simulink model "Core1MC"  (R2025a)
settings: Solver=FixedStepDiscrete  StartTime=0.0  StopTime=10.0  RelTol=1e-3
settings Model: Creator=mfussi  LastModifiedBy=mfussi
settings OptimizationCC: DefaultParameterBehavior=Inlined  EnhancedBackFolding=on  PassReuseOutputArgsAs=Individual arguments  ZeroExternalMemoryAtStartup=off  ZeroInternalMemoryAtStartup=off  OptimizeBlockOrder=speed  DifferentSizesBufferReuse=on  OptimizationCustomize=off  EfficientTunableParamExpr=on
settings DebuggingCC: ParameterTunabilityLossMsg=error
settings SFSimCC: MATLABDynamicMemAlloc=off
settings RTWCC: SystemTargetFile=ert.tlc  TemplateMakefile=ert_default_tmf  Description=Embedded Coder
settings CodeAppCC: ForceParamTrailComments=on  IgnoreCustomStorageClasses=off  OperatorAnnotations=on  SimulinkDataObjDesc=on  SFDataObjDesc=on  InsertBlockDesc=on
settings ERTTargetCC: ExtModeTransport=0.0  ExtModeStaticAlloc=off  ExtModeMexFile=ext_comm  ExtModeIntrfLevel=Level1  ERTCustomFileTemplate=example_file_process.tlc  TargetLangStandard=C99 (ISO)  GenerateSampleERTMain=on

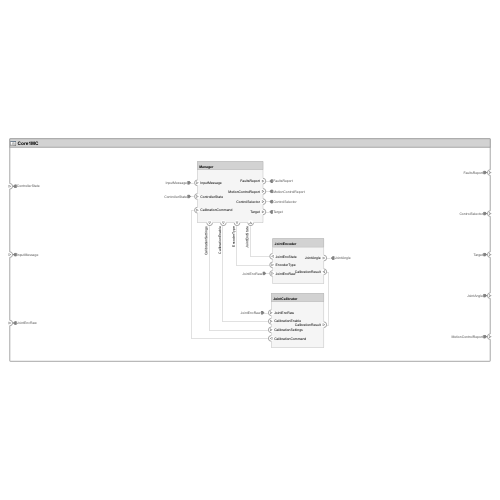
[thumbnail: Simulink's stored preview of the top-level diagram]
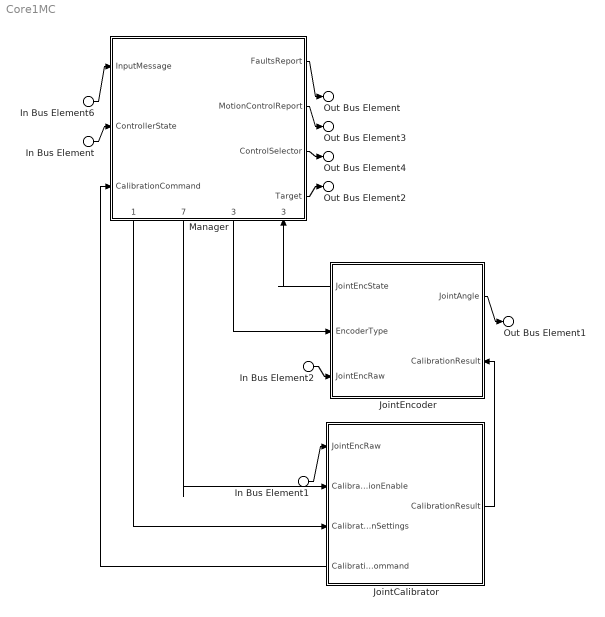
== system Core1MC ==
  In Bus Element : Inport  PortName=ControllerState
  In Bus Element6 : Inport  Port=2  PortName=InputMessage
  In Bus Element2 : Inport  Port=3  PortName=JointEncRaw
  In Bus Element1 : Inport  Port=3  PortName=JointEncRaw
  JointCalibrator : Subsystem
      settings: PortSchema="{\"entries\":[{\"content\":{\"headerSize\":26,\"margin\":15,\"minimumSpacing\":25,\"sides\":[{\"content\":{\"connectorIds\":[\"In3\",\"In1\",\"In2\",\"Out2\"]},\"type\":\"ConnectorPlacement.EquallySpacedRectSide\",\"uuid\":\"01a9f67f-de41-4770-8c99-b8ecc5be53ce\"},{\"content\":{\"connectorIds\":[\"Out1\"],\"side\":\"RIGHT\"},\"type\":\"ConnectorPlacement.EquallySpacedRectSide\",\"uuid\":\"bf951eb2-be85-4331-ab1b-e1ec4c58de10\"},{\"content\":{\"side\":\"TOP\"},\"type\":\"ConnectorPlacement.EquallySpacedRectSide\",\"uuid\":\"bda0090a-3dbc-4c35-be89-fb46a9401bc0\"},{\"content\":{\"side\":\"BOTTOM\"},\"type\":\"ConnectorPlacement.EquallySpacedRectSide\",\"uuid\":\"ec3dea10-cab4-440e-89eb-654eef2537c3\"}]},\"type\":\"ConnectorPlacement.EquallySpacedConnector\",\"uuid\":\"c83d3565-87fc-4d8e-ad9f-6c471e7c3840\"}],\"packageUris\":[\"http://schema.mathworks.com/mf0/Connector/R2020b\"],\"version\":\"1.0\"}"
  JointEncoder : Subsystem
      settings: PortSchema="{\"entries\":[{\"content\":{\"headerSize\":26,\"margin\":15,\"minimumSpacing\":25,\"sides\":[{\"content\":{\"connectorIds\":[\"Out1\",\"In1\",\"In3\"]},\"type\":\"ConnectorPlacement.EquallySpacedRectSide\",\"uuid\":\"01a9f67f-de41-4770-8c99-b8ecc5be53ce\"},{\"content\":{\"connectorIds\":[\"Out2\",\"In2\"],\"side\":\"RIGHT\"},\"type\":\"ConnectorPlacement.EquallySpacedRectSide\",\"uuid\":\"bf951eb2-be85-4331-ab1b-e1ec4c58de10\"},{\"content\":{\"side\":\"TOP\"},\"type\":\"ConnectorPlacement.EquallySpacedRectSide\",\"uuid\":\"bda0090a-3dbc-4c35-be89-fb46a9401bc0\"},{\"content\":{\"side\":\"BOTTOM\"},\"type\":\"ConnectorPlacement.EquallySpacedRectSide\",\"uuid\":\"08402c68-e81a-4e51-a9bb-186315986595\"}]},\"type\":\"ConnectorPlacement.EquallySpacedConnector\",\"uuid\":\"c83d3565-87fc-4d8e-ad9f-6c471e7c3840\"}],\"packageUris\":[\"http://schema.mathworks.com/mf0/Connector/R2020b\"],\"version\":\"1.0\"}"
  Manager : Subsystem
      settings: PortSchema="{\"entries\":[{\"content\":{\"headerSize\":26,\"margin\":15,\"minimumSpacing\":25,\"sides\":[{\"content\":{\"connectorIds\":[\"In1\",\"In4\",\"In2\"]},\"type\":\"ConnectorPlacement.EquallySpacedRectSide\",\"uuid\":\"8e6109ac-b489-4864-8b2b-7ebf0beccfe4\"},{\"content\":{\"connectorIds\":[\"Out2\",\"Out5\",\"Out4\",\"Out6\"],\"side\":\"RIGHT\"},\"type\":\"ConnectorPlacement.EquallySpacedRectSide\",\"uuid\":\"71828a7e-6b05-4f57-abc1-6f865453b9f6\"},{\"content\":{\"side\":\"TOP\"},\"type\":\"ConnectorPlacement.EquallySpacedRectSide\",\"uuid\":\"bfeeaaf9-6170-4b48-807f-b679c72692dc\"},{\"content\":{\"connectorIds\":[\"Out1\",\"Out7\",\"Out3\",\"In3\"],\"side\":\"BOTTOM\"},\"type\":\"ConnectorPlacement.EquallySpacedRectSide\",\"uuid\":\"8d96d7f2-73a1-4d5a-99fb-90680abef3dc\"}]},\"type\":\"ConnectorPlacement.EquallySpacedConnector\",\"uuid\":\"352ed8e9-1880-4bea-97e7-a2aba6f573a0\"}],\"packageUris\":[\"http://schema.mathworks.com/mf0/Connector/R2020b\"],\"version\":\"1.0\"}"
  Out Bus Element : Outport  PortName=FaultsReport
  Out Bus Element4 : Outport  Port=2  PortName=ControlSelector
  Out Bus Element2 : Outport  Port=3  PortName=Target
  Out Bus Element1 : Outport  Port=4  PortName=JointAngle
  Out Bus Element3 : Outport  Port=5  PortName=MotionControlReport
  wires:
  Manager/7(CalibrationEnable) -> JointCalibrator/1(CalibrationEnable)
  Manager/6(Target) -> Out Bus Element2/1
  Manager/1(CalibrationSettings) -> JointCalibrator/2(CalibrationSettings)
  JointEncoder/2(JointAngle) -> Out Bus Element1/1
  In Bus Element2/1 -> JointEncoder/3(JointEncRaw)
  Manager/2(FaultsReport) -> Out Bus Element/1
  JointCalibrator/2(CalibrationCommand) -> Manager/2(CalibrationCommand)
  Manager/5(MotionControlReport) -> Out Bus Element3/1
  In Bus Element1/1 -> JointCalibrator/3(JointEncRaw)
  Manager/3(EncoderType) -> JointEncoder/1(EncoderType)
  In Bus Element6/1 -> Manager/1(InputMessage)
  JointCalibrator/1(CalibrationResult) -> JointEncoder/2(CalibrationResult)
  JointEncoder/1(JointEncState) -> Manager/3(JointEncState)
  Manager/4(ControlSelector) -> Out Bus Element4/1
  In Bus Element/1 -> Manager/4(ControllerState)

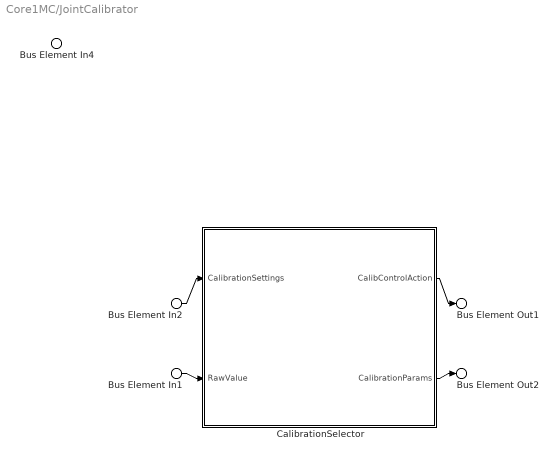
== system Core1MC/JointCalibrator ==
  Bus Element In4 : Inport  PortName=CalibrationEnable
  Bus Element In2 : Inport  Port=2  PortName=CalibrationSettings
  Bus Element In1 : Inport  Port=3  PortName=JointEncRaw
  CalibrationSelector : Subsystem
      settings: PortSchema="{\"entries\":[{\"content\":{\"headerSize\":26,\"margin\":15,\"minimumSpacing\":25,\"sides\":[{\"content\":{\"connectorIds\":[\"In1\",\"In2\"]},\"type\":\"ConnectorPlacement.EquallySpacedRectSide\",\"uuid\":\"8e6109ac-b489-4864-8b2b-7ebf0beccfe4\"},{\"content\":{\"connectorIds\":[\"Out1\",\"Out2\"],\"side\":\"RIGHT\"},\"type\":\"ConnectorPlacement.EquallySpacedRectSide\",\"uuid\":\"71828a7e-6b05-4f57-abc1-6f865453b9f6\"},{\"content\":{\"side\":\"TOP\"},\"type\":\"ConnectorPlacement.EquallySpacedRectSide\",\"uuid\":\"bfeeaaf9-6170-4b48-807f-b679c72692dc\"},{\"content\":{\"side\":\"BOTTOM\"},\"type\":\"ConnectorPlacement.EquallySpacedRectSide\",\"uuid\":\"25c92704-7839-4043-9d29-39ffe7db8a81\"}]},\"type\":\"ConnectorPlacement.EquallySpacedConnector\",\"uuid\":\"352ed8e9-1880-4bea-97e7-a2aba6f573a0\"}],\"packageUris\":[\"http://schema.mathworks.com/mf0/Connector/R2020b\"],\"version\":\"1.0\"}"
  Bus Element Out2 : Outport  PortName=CalibrationResult
  Bus Element Out1 : Outport  Port=2  PortName=CalibrationCommand
  wires:
  Bus Element In2/1 -> CalibrationSelector/1(CalibrationSettings)
  CalibrationSelector/2(CalibrationParams) -> Bus Element Out2/1
  Bus Element In1/1 -> CalibrationSelector/2(RawValue)
  CalibrationSelector/1(CalibControlAction) -> Bus Element Out1/1

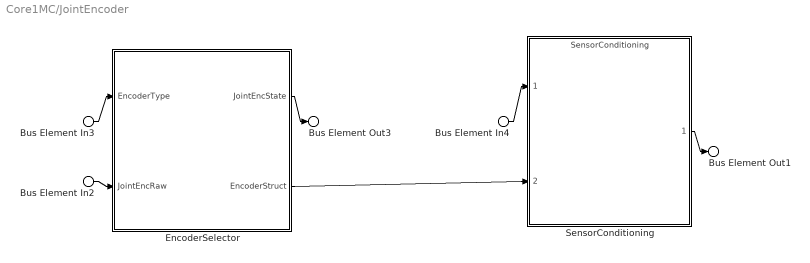
== system Core1MC/JointEncoder ==
  Bus Element In3 : Inport  PortName=EncoderType
  Bus Element In4 : Inport  Port=2  PortName=CalibrationResult
  Bus Element In2 : Inport  Port=3  PortName=JointEncRaw
  EncoderSelector : Subsystem
      settings: PortSchema="{\"entries\":[{\"content\":{\"headerSize\":26,\"margin\":15,\"minimumSpacing\":25,\"sides\":[{\"content\":{\"connectorIds\":[\"In1\",\"In2\"]},\"type\":\"ConnectorPlacement.EquallySpacedRectSide\",\"uuid\":\"8f52fc44-033b-42c5-ba74-e10c3c4c9620\"},{\"content\":{\"connectorIds\":[\"Out1\",\"Out2\"],\"side\":\"RIGHT\"},\"type\":\"ConnectorPlacement.EquallySpacedRectSide\",\"uuid\":\"3378411c-333a-4ac7-97cd-fc73e032020d\"},{\"content\":{\"side\":\"TOP\"},\"type\":\"ConnectorPlacement.EquallySpacedRectSide\",\"uuid\":\"71f34e7e-b8af-4493-b4da-76896ccc3fbc\"}]},\"type\":\"ConnectorPlacement.EquallySpacedConnector\",\"uuid\":\"3896a3b2-2849-4eb4-a68e-00b6690583b8\"}],\"packageUris\":[\"http://schema.mathworks.com/mf0/Connector/R2020b\"],\"version\":\"1.0\"}"
  SensorConditioning : ModelReference  ModelNameDialog=SensorConditioning.slx  SimulationMode=Normal  ScheduleRates=on  ModelReferenceVersion=1.2
      settings: PortSchema="{\"entries\":[{\"content\":{\"headerSize\":38,\"margin\":15,\"minimumSpacing\":25,\"sides\":[{\"content\":{\"connectorIds\":[\"In1\",\"In2\"]},\"type\":\"ConnectorPlacement.EquallySpacedRectSide\",\"uuid\":\"6d6857fa-f5c9-43b4-a306-0920391a2fd0\"},{\"content\":{\"connectorIds\":[\"Out1\"],\"side\":\"RIGHT\"},\"type\":\"ConnectorPlacement.EquallySpacedRectSide\",\"uuid\":\"4567897e-6982-4f2c-af43-5ed4bc8792a2\"},{\"content\":{\"side\":\"TOP\"},\"type\":\"ConnectorPlacement.EquallySpacedRectSide\",\"uuid\":\"b9101744-fe35-433d-bb4c-e7449aefab81\"}]},\"type\":\"ConnectorPlacement.EquallySpacedConnector\",\"uuid\":\"96c92cf5-557b-4ff0-b6b4-f2ae6063b6b3\"}],\"packageUris\":[\"http://schema.mathworks.com/mf0/Connector/R2020b\"],\"version\":\"1.0\"}"
  Bus Element Out3 : Outport  PortName=JointEncState
  Bus Element Out1 : Outport  Port=2  PortName=JointAngle
  wires:
  Bus Element In3/1 -> EncoderSelector/1(EncoderType)
  SensorConditioning/1 -> Bus Element Out1/1
  Bus Element In4/1 -> SensorConditioning/1
  Bus Element In2/1 -> EncoderSelector/2(JointEncRaw)
  EncoderSelector/2(EncoderStruct) -> SensorConditioning/2
  EncoderSelector/1(JointEncState) -> Bus Element Out3/1

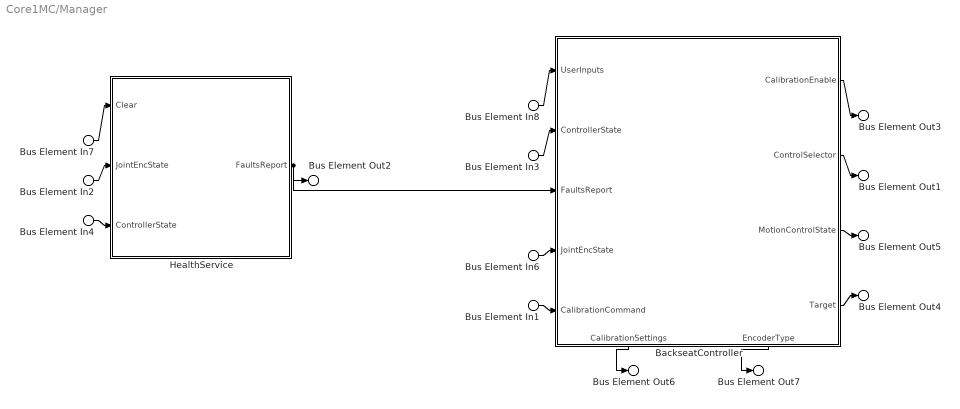
== system Core1MC/Manager ==
  Bus Element In8 : Inport  PortName=InputMessage
  Bus Element In7 : Inport  PortName=InputMessage  Element=ClearFaults
  Bus Element In1 : Inport  Port=2  PortName=CalibrationCommand
  Bus Element In2 : Inport  Port=3  PortName=JointEncState
  Bus Element In6 : Inport  Port=3  PortName=JointEncState
  Bus Element In3 : Inport  Port=4  PortName=ControllerState
  Bus Element In4 : Inport  Port=4  PortName=ControllerState
  "BackseatController   " : Subsystem
      settings: PortSchema="{\"entries\":[{\"content\":{\"headerSize\":26,\"margin\":15,\"minimumSpacing\":25,\"sides\":[{\"content\":{\"connectorIds\":[\"In1\",\"In2\",\"In4\",\"In3\",\"In5\"]},\"type\":\"ConnectorPlacement.EquallySpacedRectSide\",\"uuid\":\"85ee84b9-0970-40ce-bfce-e5d9bdcbaee5\"},{\"content\":{\"connectorIds\":[\"Out4\",\"Out3\",\"Out5\",\"Out6\"],\"side\":\"RIGHT\"},\"type\":\"ConnectorPlacement.EquallySpacedRectSide\",\"uuid\":\"4b841b97-ee1a-48ec-855b-c93d07f120e6\"},{\"content\":{\"side\":\"TOP\"},\"type\":\"ConnectorPlacement.EquallySpacedRectSide\",\"uuid\":\"7d8ccfe4-6449-46f0-b4fc-bdc759f5a65a\"},{\"content\":{\"connectorIds\":[\"Out1\",\"Out2\"],\"side\":\"BOTTOM\"},\"type\":\"ConnectorPlacement.EquallySpacedRectSide\",\"uuid\":\"0ea367ec-c1df-4801-a6d0-378c12bf5467\"}]},\"type\":\"ConnectorPlacement.EquallySpacedConnector\",\"uuid\":\"5fa6d4b4-3693-4e78-8a63-6d39a883b60e\"}],\"packageUris\":[\"http://schema.mathworks.com/mf0/Connector/R2020b\"],\"version\":\"1.0\"}"
  HealthService : Subsystem
      settings: PortSchema="{\"entries\":[{\"content\":{\"headerSize\":26,\"margin\":15,\"minimumSpacing\":25,\"sides\":[{\"content\":{\"connectorIds\":[\"In1\",\"In2\",\"In3\"]},\"type\":\"ConnectorPlacement.EquallySpacedRectSide\",\"uuid\":\"85ee84b9-0970-40ce-bfce-e5d9bdcbaee5\"},{\"content\":{\"connectorIds\":[\"Out1\"],\"side\":\"RIGHT\"},\"type\":\"ConnectorPlacement.EquallySpacedRectSide\",\"uuid\":\"4b841b97-ee1a-48ec-855b-c93d07f120e6\"},{\"content\":{\"side\":\"TOP\"},\"type\":\"ConnectorPlacement.EquallySpacedRectSide\",\"uuid\":\"7d8ccfe4-6449-46f0-b4fc-bdc759f5a65a\"}]},\"type\":\"ConnectorPlacement.EquallySpacedConnector\",\"uuid\":\"5fa6d4b4-3693-4e78-8a63-6d39a883b60e\"}],\"packageUris\":[\"http://schema.mathworks.com/mf0/Connector/R2020b\"],\"version\":\"1.0\"}"
  Bus Element Out6 : Outport  PortName=CalibrationSettings
  Bus Element Out2 : Outport  Port=2  PortName=FaultsReport
  Bus Element Out7 : Outport  Port=3  PortName=EncoderType
  Bus Element Out1 : Outport  Port=4  PortName=ControlSelector
  Bus Element Out5 : Outport  Port=5  PortName=MotionControlReport
  Bus Element Out4 : Outport  Port=6  PortName=Target
  Bus Element Out3 : Outport  Port=7  PortName=CalibrationEnable
  wires:
  "BackseatController   "/4(CalibrationEnable) -> Bus Element Out3/1
  "BackseatController   "/3(ControlSelector) -> Bus Element Out1/1
  Bus Element In3/1 -> "BackseatController   "/2(ControllerState)
  HealthService/1(FaultsReport) -> "BackseatController   "/4(FaultsReport), Bus Element Out2/1
  Bus Element In2/1 -> HealthService/2(JointEncState)
  Bus Element In4/1 -> HealthService/3(ControllerState)
  Bus Element In6/1 -> "BackseatController   "/3(JointEncState)
  "BackseatController   "/5(MotionControlState) -> Bus Element Out5/1
  Bus Element In7/1 -> HealthService/1(Clear)
  Bus Element In8/1 -> "BackseatController   "/1(UserInputs)
  "BackseatController   "/6(Target) -> Bus Element Out4/1
  "BackseatController   "/2(EncoderType) -> Bus Element Out7/1
  Bus Element In1/1 -> "BackseatController   "/5(CalibrationCommand)
  "BackseatController   "/1(CalibrationSettings) -> Bus Element Out6/1

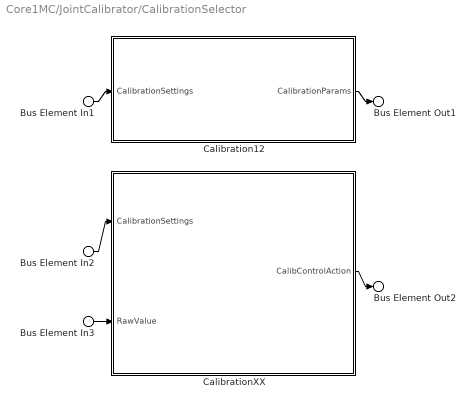
== system Core1MC/JointCalibrator/CalibrationSelector ==
  Bus Element In1 : Inport  PortName=CalibrationSettings
  Bus Element In2 : Inport  PortName=CalibrationSettings
  Bus Element In3 : Inport  Port=2  PortName=RawValue
  Calibration12 : Subsystem
      settings: PortSchema="{\"entries\":[{\"content\":{\"headerSize\":26,\"margin\":15,\"minimumSpacing\":25,\"sides\":[{\"content\":{\"connectorIds\":[\"In1\"]},\"type\":\"ConnectorPlacement.EquallySpacedRectSide\",\"uuid\":\"8e6109ac-b489-4864-8b2b-7ebf0beccfe4\"},{\"content\":{\"connectorIds\":[\"Out1\"],\"side\":\"RIGHT\"},\"type\":\"ConnectorPlacement.EquallySpacedRectSide\",\"uuid\":\"71828a7e-6b05-4f57-abc1-6f865453b9f6\"},{\"content\":{\"side\":\"TOP\"},\"type\":\"ConnectorPlacement.EquallySpacedRectSide\",\"uuid\":\"bfeeaaf9-6170-4b48-807f-b679c72692dc\"}]},\"type\":\"ConnectorPlacement.EquallySpacedConnector\",\"uuid\":\"352ed8e9-1880-4bea-97e7-a2aba6f573a0\"}],\"packageUris\":[\"http://schema.mathworks.com/mf0/Connector/R2020b\"],\"version\":\"1.0\"}"
  CalibrationXX : Subsystem
      settings: PortSchema="{\"entries\":[{\"content\":{\"headerSize\":26,\"margin\":15,\"minimumSpacing\":25,\"sides\":[{\"content\":{\"connectorIds\":[\"In1\",\"In2\"]},\"type\":\"ConnectorPlacement.EquallySpacedRectSide\",\"uuid\":\"8e6109ac-b489-4864-8b2b-7ebf0beccfe4\"},{\"content\":{\"connectorIds\":[\"Out1\"],\"side\":\"RIGHT\"},\"type\":\"ConnectorPlacement.EquallySpacedRectSide\",\"uuid\":\"71828a7e-6b05-4f57-abc1-6f865453b9f6\"},{\"content\":{\"side\":\"TOP\"},\"type\":\"ConnectorPlacement.EquallySpacedRectSide\",\"uuid\":\"bfeeaaf9-6170-4b48-807f-b679c72692dc\"},{\"content\":{\"side\":\"BOTTOM\"},\"type\":\"ConnectorPlacement.EquallySpacedRectSide\",\"uuid\":\"376d2493-7fe7-4dcb-93f0-7b1cd430ade4\"}]},\"type\":\"ConnectorPlacement.EquallySpacedConnector\",\"uuid\":\"352ed8e9-1880-4bea-97e7-a2aba6f573a0\"}],\"packageUris\":[\"http://schema.mathworks.com/mf0/Connector/R2020b\"],\"version\":\"1.0\"}"
  Bus Element Out2 : Outport  PortName=CalibControlAction
  Bus Element Out1 : Outport  Port=2  PortName=CalibrationParams
  wires:
  Bus Element In1/1 -> Calibration12/1(CalibrationSettings)
  Calibration12/1(CalibrationParams) -> Bus Element Out1/1
  Bus Element In2/1 -> CalibrationXX/1(CalibrationSettings)
  Bus Element In3/1 -> CalibrationXX/2(RawValue)
  CalibrationXX/1(CalibControlAction) -> Bus Element Out2/1

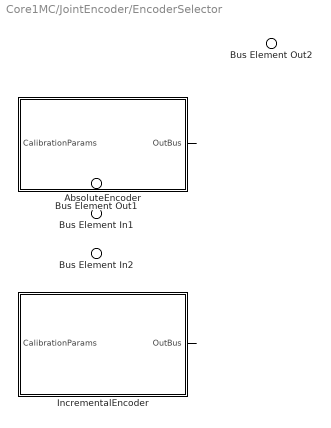
== system Core1MC/JointEncoder/EncoderSelector ==
  Bus Element In1 : Inport  PortName=EncoderType
  Bus Element In2 : Inport  Port=2  PortName=JointEncRaw
  AbsoluteEncoder : Subsystem
      settings: PortSchema="{\"entries\":[{\"content\":{\"headerSize\":26,\"margin\":15,\"minimumSpacing\":25,\"sides\":[{\"content\":{\"connectorIds\":[\"In1\"]},\"type\":\"ConnectorPlacement.EquallySpacedRectSide\",\"uuid\":\"8e6109ac-b489-4864-8b2b-7ebf0beccfe4\"},{\"content\":{\"connectorIds\":[\"Out1\"],\"side\":\"RIGHT\"},\"type\":\"ConnectorPlacement.EquallySpacedRectSide\",\"uuid\":\"71828a7e-6b05-4f57-abc1-6f865453b9f6\"},{\"content\":{\"side\":\"TOP\"},\"type\":\"ConnectorPlacement.EquallySpacedRectSide\",\"uuid\":\"bfeeaaf9-6170-4b48-807f-b679c72692dc\"}]},\"type\":\"ConnectorPlacement.EquallySpacedConnector\",\"uuid\":\"352ed8e9-1880-4bea-97e7-a2aba6f573a0\"}],\"packageUris\":[\"http://schema.mathworks.com/mf0/Connector/R2020b\"],\"version\":\"1.0\"}"
  IncrementalEncoder : Subsystem
      settings: PortSchema="{\"entries\":[{\"content\":{\"headerSize\":26,\"margin\":15,\"minimumSpacing\":25,\"sides\":[{\"content\":{\"connectorIds\":[\"In1\"]},\"type\":\"ConnectorPlacement.EquallySpacedRectSide\",\"uuid\":\"8e6109ac-b489-4864-8b2b-7ebf0beccfe4\"},{\"content\":{\"connectorIds\":[\"Out1\"],\"side\":\"RIGHT\"},\"type\":\"ConnectorPlacement.EquallySpacedRectSide\",\"uuid\":\"71828a7e-6b05-4f57-abc1-6f865453b9f6\"},{\"content\":{\"side\":\"TOP\"},\"type\":\"ConnectorPlacement.EquallySpacedRectSide\",\"uuid\":\"bfeeaaf9-6170-4b48-807f-b679c72692dc\"},{\"content\":{\"side\":\"BOTTOM\"},\"type\":\"ConnectorPlacement.EquallySpacedRectSide\",\"uuid\":\"a15bd14f-14b1-4784-ba04-128ef95cb1ea\"}]},\"type\":\"ConnectorPlacement.EquallySpacedConnector\",\"uuid\":\"352ed8e9-1880-4bea-97e7-a2aba6f573a0\"}],\"packageUris\":[\"http://schema.mathworks.com/mf0/Connector/R2020b\"],\"version\":\"1.0\"}"
  Bus Element Out2 : Outport  PortName=JointEncState
  Bus Element Out1 : Outport  Port=2  PortName=EncoderStruct
  wires:
  AbsoluteEncoder/1(OutBus) -> ?
  IncrementalEncoder/1(OutBus) -> ?

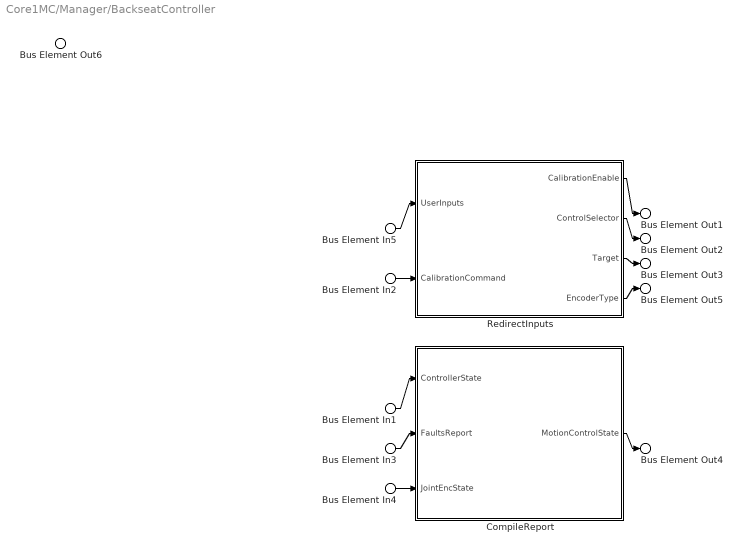
== system Core1MC/Manager/BackseatController    ==
  Bus Element In5 : Inport  PortName=UserInputs
  Bus Element In1 : Inport  Port=2  PortName=ControllerState
  Bus Element In4 : Inport  Port=3  PortName=JointEncState
  Bus Element In3 : Inport  Port=4  PortName=FaultsReport
  Bus Element In2 : Inport  Port=5  PortName=CalibrationCommand
  CompileReport : Subsystem
      settings: PortSchema="{\"entries\":[{\"content\":{\"headerSize\":26,\"margin\":15,\"minimumSpacing\":25,\"sides\":[{\"content\":{\"connectorIds\":[\"In1\",\"In2\",\"In3\"]},\"type\":\"ConnectorPlacement.EquallySpacedRectSide\",\"uuid\":\"b721ea92-b23b-49c6-b256-e109cfde6d9a\"},{\"content\":{\"connectorIds\":[\"Out1\"],\"side\":\"RIGHT\"},\"type\":\"ConnectorPlacement.EquallySpacedRectSide\",\"uuid\":\"01ecff02-faf6-44fc-85cd-eb338f239b8b\"},{\"content\":{\"side\":\"TOP\"},\"type\":\"ConnectorPlacement.EquallySpacedRectSide\",\"uuid\":\"b7f583c7-535b-43ea-9e2b-1d6295f5e2cc\"}]},\"type\":\"ConnectorPlacement.EquallySpacedConnector\",\"uuid\":\"374a74ae-7551-4f3a-8e98-a33b88a70ffb\"}],\"packageUris\":[\"http://schema.mathworks.com/mf0/Connector/R2020b\"],\"version\":\"1.0\"}"
  RedirectInputs : Subsystem
      settings: PortSchema="{\"entries\":[{\"content\":{\"headerSize\":26,\"margin\":15,\"minimumSpacing\":25,\"sides\":[{\"content\":{\"connectorIds\":[\"In1\",\"In2\"]},\"type\":\"ConnectorPlacement.EquallySpacedRectSide\",\"uuid\":\"b721ea92-b23b-49c6-b256-e109cfde6d9a\"},{\"content\":{\"connectorIds\":[\"Out1\",\"Out2\",\"Out3\",\"Out4\"],\"side\":\"RIGHT\"},\"type\":\"ConnectorPlacement.EquallySpacedRectSide\",\"uuid\":\"01ecff02-faf6-44fc-85cd-eb338f239b8b\"},{\"content\":{\"side\":\"TOP\"},\"type\":\"ConnectorPlacement.EquallySpacedRectSide\",\"uuid\":\"b7f583c7-535b-43ea-9e2b-1d6295f5e2cc\"}]},\"type\":\"ConnectorPlacement.EquallySpacedConnector\",\"uuid\":\"374a74ae-7551-4f3a-8e98-a33b88a70ffb\"}],\"packageUris\":[\"http://schema.mathworks.com/mf0/Connector/R2020b\"],\"version\":\"1.0\"}"
  Bus Element Out6 : Outport  PortName=CalibrationSettings
  Bus Element Out5 : Outport  Port=2  PortName=EncoderType
  Bus Element Out2 : Outport  Port=3  PortName=ControlSelector
  Bus Element Out1 : Outport  Port=4  PortName=CalibrationEnable
  Bus Element Out4 : Outport  Port=5  PortName=MotionControlState
  Bus Element Out3 : Outport  Port=6  PortName=Target
  wires:
  CompileReport/1(MotionControlState) -> Bus Element Out4/1
  Bus Element In4/1 -> CompileReport/3(JointEncState)
  Bus Element In3/1 -> CompileReport/2(FaultsReport)
  Bus Element In1/1 -> CompileReport/1(ControllerState)
  Bus Element In5/1 -> RedirectInputs/1(UserInputs)
  RedirectInputs/3(Target) -> Bus Element Out3/1
  RedirectInputs/2(ControlSelector) -> Bus Element Out2/1
  RedirectInputs/1(CalibrationEnable) -> Bus Element Out1/1
  Bus Element In2/1 -> RedirectInputs/2(CalibrationCommand)
  RedirectInputs/4(EncoderType) -> Bus Element Out5/1

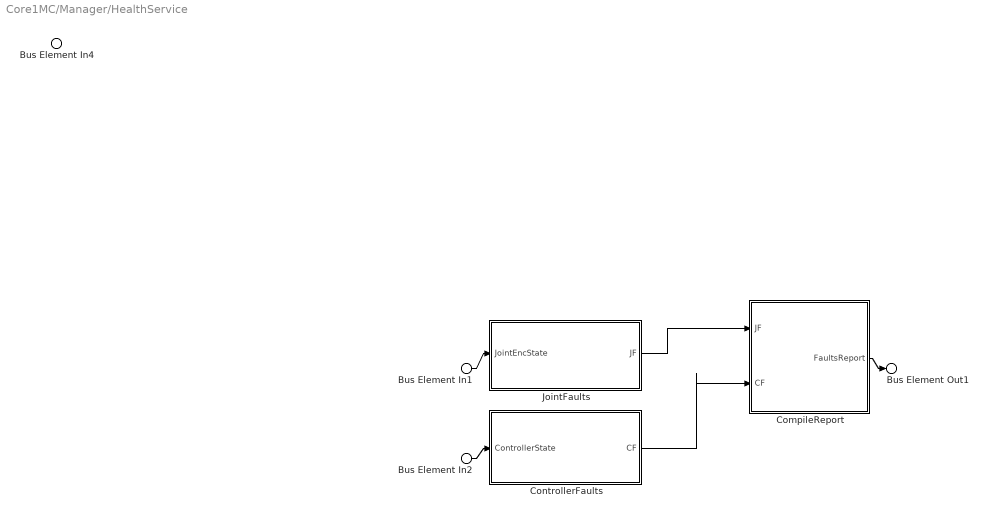
== system Core1MC/Manager/HealthService ==
  Bus Element In4 : Inport  PortName=Clear
  Bus Element In1 : Inport  Port=2  PortName=JointEncState
  Bus Element In2 : Inport  Port=3  PortName=ControllerState
  CompileReport : Subsystem
      settings: PortSchema="{\"entries\":[{\"content\":{\"headerSize\":26,\"margin\":15,\"minimumSpacing\":25,\"sides\":[{\"content\":{\"connectorIds\":[\"In1\",\"In2\"]},\"type\":\"ConnectorPlacement.EquallySpacedRectSide\",\"uuid\":\"85ee84b9-0970-40ce-bfce-e5d9bdcbaee5\"},{\"content\":{\"connectorIds\":[\"Out1\"],\"side\":\"RIGHT\"},\"type\":\"ConnectorPlacement.EquallySpacedRectSide\",\"uuid\":\"4b841b97-ee1a-48ec-855b-c93d07f120e6\"},{\"content\":{\"side\":\"TOP\"},\"type\":\"ConnectorPlacement.EquallySpacedRectSide\",\"uuid\":\"7d8ccfe4-6449-46f0-b4fc-bdc759f5a65a\"}]},\"type\":\"ConnectorPlacement.EquallySpacedConnector\",\"uuid\":\"5fa6d4b4-3693-4e78-8a63-6d39a883b60e\"}],\"packageUris\":[\"http://schema.mathworks.com/mf0/Connector/R2020b\"],\"version\":\"1.0\"}"
  ControllerFaults : Subsystem
      settings: PortSchema="{\"entries\":[{\"content\":{\"headerSize\":26,\"margin\":15,\"minimumSpacing\":25,\"sides\":[{\"content\":{\"connectorIds\":[\"In1\"]},\"type\":\"ConnectorPlacement.EquallySpacedRectSide\",\"uuid\":\"85ee84b9-0970-40ce-bfce-e5d9bdcbaee5\"},{\"content\":{\"connectorIds\":[\"Out1\"],\"side\":\"RIGHT\"},\"type\":\"ConnectorPlacement.EquallySpacedRectSide\",\"uuid\":\"4b841b97-ee1a-48ec-855b-c93d07f120e6\"},{\"content\":{\"side\":\"TOP\"},\"type\":\"ConnectorPlacement.EquallySpacedRectSide\",\"uuid\":\"7d8ccfe4-6449-46f0-b4fc-bdc759f5a65a\"}]},\"type\":\"ConnectorPlacement.EquallySpacedConnector\",\"uuid\":\"5fa6d4b4-3693-4e78-8a63-6d39a883b60e\"}],\"packageUris\":[\"http://schema.mathworks.com/mf0/Connector/R2020b\"],\"version\":\"1.0\"}"
  JointFaults : Subsystem
      settings: PortSchema="{\"entries\":[{\"content\":{\"headerSize\":26,\"margin\":15,\"minimumSpacing\":25,\"sides\":[{\"content\":{\"connectorIds\":[\"In1\"]},\"type\":\"ConnectorPlacement.EquallySpacedRectSide\",\"uuid\":\"85ee84b9-0970-40ce-bfce-e5d9bdcbaee5\"},{\"content\":{\"connectorIds\":[\"Out1\"],\"side\":\"RIGHT\"},\"type\":\"ConnectorPlacement.EquallySpacedRectSide\",\"uuid\":\"4b841b97-ee1a-48ec-855b-c93d07f120e6\"},{\"content\":{\"side\":\"TOP\"},\"type\":\"ConnectorPlacement.EquallySpacedRectSide\",\"uuid\":\"7d8ccfe4-6449-46f0-b4fc-bdc759f5a65a\"}]},\"type\":\"ConnectorPlacement.EquallySpacedConnector\",\"uuid\":\"5fa6d4b4-3693-4e78-8a63-6d39a883b60e\"}],\"packageUris\":[\"http://schema.mathworks.com/mf0/Connector/R2020b\"],\"version\":\"1.0\"}"
  Bus Element Out1 : Outport  PortName=FaultsReport
  wires:
  Bus Element In1/1 -> JointFaults/1(JointEncState)
  Bus Element In2/1 -> ControllerFaults/1(ControllerState)
  JointFaults/1(JF) -> CompileReport/1(JF)
  ControllerFaults/1(CF) -> CompileReport/2(CF)
  CompileReport/1(FaultsReport) -> Bus Element Out1/1

== system Core1MC/JointCalibrator/CalibrationSelector/Calibration12 ==
  Bus Element In1 : Inport  PortName=CalibrationSettings
  Bus Element Out1 : Outport  PortName=CalibrationParams

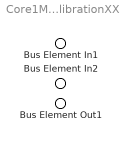
== system Core1MC/JointCalibrator/CalibrationSelector/CalibrationXX ==
  Bus Element In1 : Inport  PortName=CalibrationSettings
  Bus Element In2 : Inport  Port=2  PortName=RawValue
  Bus Element Out1 : Outport  PortName=CalibControlAction

== system Core1MC/JointEncoder/EncoderSelector/AbsoluteEncoder ==
  Bus Element In1 : Inport  PortName=CalibrationParams
  Bus Element Out1 : Outport  PortName=OutBus

== system Core1MC/JointEncoder/EncoderSelector/IncrementalEncoder ==
  Bus Element In1 : Inport  PortName=CalibrationParams
  Bus Element Out1 : Outport  PortName=OutBus

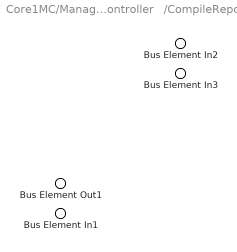
== system Core1MC/Manager/BackseatController   /CompileReport ==
  Bus Element In3 : Inport  PortName=ControllerState
  Bus Element In2 : Inport  Port=2  PortName=FaultsReport
  Bus Element In1 : Inport  Port=3  PortName=JointEncState
  Bus Element Out1 : Outport  PortName=MotionControlState

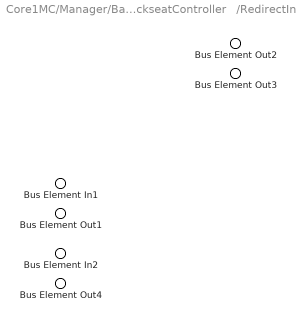
== system Core1MC/Manager/BackseatController   /RedirectInputs ==
  Bus Element In1 : Inport  PortName=UserInputs
  Bus Element In2 : Inport  Port=2  PortName=CalibrationCommand
  Bus Element Out3 : Outport  PortName=CalibrationEnable
  Bus Element Out2 : Outport  Port=2  PortName=ControlSelector
  Bus Element Out1 : Outport  Port=3  PortName=Target
  Bus Element Out4 : Outport  Port=4  PortName=EncoderType

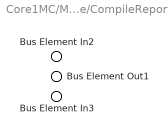
== system Core1MC/Manager/HealthService/CompileReport ==
  Bus Element In2 : Inport  PortName=JF
  Bus Element In3 : Inport  Port=2  PortName=CF
  Bus Element Out1 : Outport  PortName=FaultsReport

== system Core1MC/Manager/HealthService/ControllerFaults ==
  Bus Element In1 : Inport  PortName=ControllerState
  Bus Element Out1 : Outport  PortName=CF

== system Core1MC/Manager/HealthService/JointFaults ==
  Bus Element In1 : Inport  PortName=JointEncState
  Bus Element Out1 : Outport  PortName=JF
